simulink model "MSICA_Projet1_StructureSansControle"  (R2018a)
settings: Solver=VariableStepAuto  StartTime=0.0  StopTime=10.0  RelTol=1e-3
values from neighbouring files (symbols this model uses):
  A_S1_S2 = [ zeros(3,3) eye(3) ... (first row only)    [DonneesProjet.m]
  A_S2_S3 = [ zeros(3,3) eye(3) ... (first row only)    [DonneesProjet.m]
  B_S1_S2 = [zeros(3,3); inv(M_S1_S2)]    [DonneesProjet.m]
  B_S2_S3 = [zeros(3,3); inv(M_S2_S3)]    [DonneesProjet.m]
  C1 = [eye(3) zeros(3,3)]    [DonneesProjet.m]
settings Model: Creator=natha  LastModifiedBy=natha
settings DataIOCC: ReturnWorkspaceOutputs=on
settings SFSimCC: SimUseLocalCustomCode=on
settings RTWCC: RTWUseLocalCustomCode=on

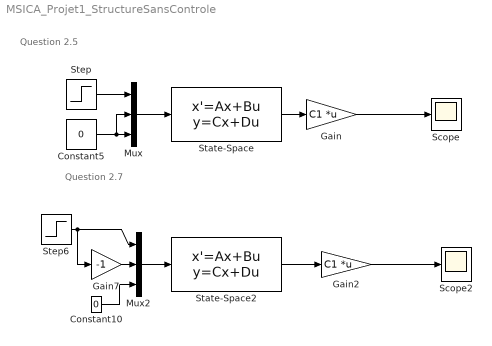
== system MSICA_Projet1_StructureSansControle ==
  note: Question 2.7
  note: Question 2.5
  Constant10 : Constant  Value=0
  Constant5 : Constant  Value=0
  Gain : Gain  Gain=C1  Multiplication=Matrix(K*u)
  Gain2 : Gain  Gain=C1  Multiplication=Matrix(K*u)
  Gain7 : Gain  Gain=-1
  Mux : Mux  Inputs=3
  Mux2 : Mux  Inputs=3
  Scope : Scope
  Scope2 : Scope
  State-Space : StateSpace  A=A_S2_S3  B=B_S2_S3  C=eye(6)  D=zeros(6,3)  InitialCondition=0
  State-Space2 : StateSpace  A=A_S1_S2  B=B_S1_S2  C=eye(6)  D=zeros(6,3)  InitialCondition=0
  Step : Step  Time=0.001  Before=100  After=0  SampleTime=0
  Step6 : Step  Time=0.001  Before=100  After=0  SampleTime=0
  wires:
  Constant5/1 -> Mux/2, Mux/3
  State-Space2/1 -> Gain2/1
  Mux/1 -> State-Space/1
  Step/1 -> Mux/1
  State-Space/1 -> Gain/1
  Gain2/1 -> Scope2/1
  Mux2/1 -> State-Space2/1
  Constant10/1 -> Mux2/3
  Gain7/1 -> Mux2/2
  Gain/1 -> Scope/1
  Step6/1 -> Mux2/1, Gain7/1
